simulink model "humanCarFollowerController_microscopic"  (R2016a)
settings: Solver=FixedStepAuto  StartTime=0.0  StopTime=inf  RelTol=1e-3
undefined symbols (not defined in the file or in its folder): Angular, Linear
libraries: robotlib x6
settings Model: Creator=ece446  LastModifiedBy=ece446
settings OptimizationCC: OptimizeModelRefInitCode=on  LifeSpan=Inf  MaxStackSize=64
settings HardwareCC: ProdBitPerInt=16  ProdBitPerPointer=16  ProdLargestAtomicFloat=None  ProdIntDivRoundTo=Undefined  ProdEndianess=Unspecified  ProdWordSize=16  ProdHWDeviceType=Generic->Unspecified (assume 32-bit Generic)  UseEmbeddedCoderFeatures=off
settings RTWCC: SystemTargetFile=ert.tlc  HardwareBoard=Robot Operating System (ROS)  TemplateMakefile=ert_default_tmf  GenerateReport=on  Toolchain=Catkin  IncludeHyperlinkInReport=on  LaunchReport=on  TargetLang=C++  GenerateTraceInfo=on  GenerateTraceReport=on  GenerateTraceReportSl=on  GenerateTraceReportSf=on  GenerateTraceReportEml=on
settings CodeAppCC: ForceParamTrailComments=on  IgnoreCustomStorageClasses=off  OperatorAnnotations=on  SimulinkDataObjDesc=on  SFDataObjDesc=on  MATLABFcnDesc=on  InsertBlockDesc=on  MATLABSourceComments=on
settings ERTTargetCC: SupportNonInlinedSFcns=on

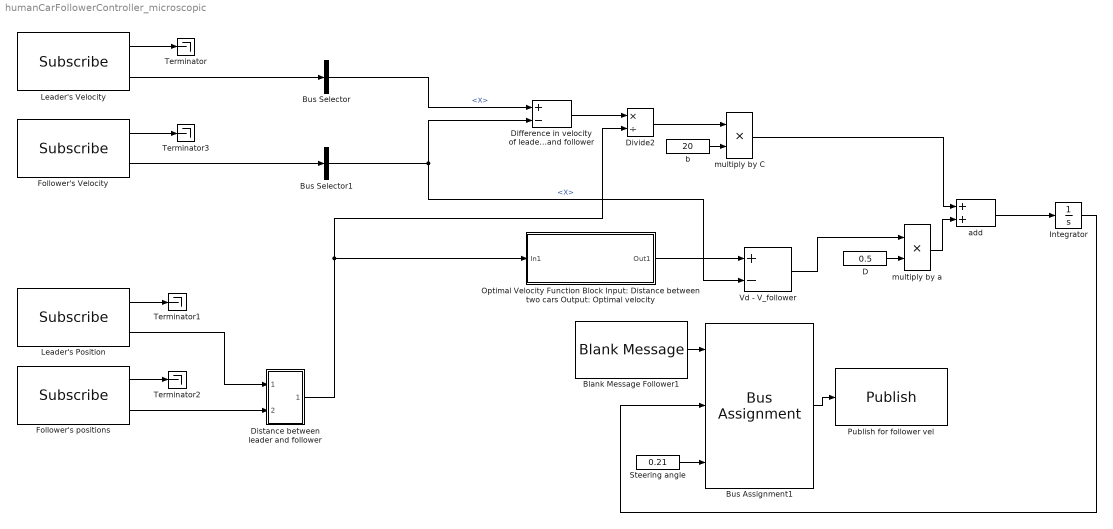
== system humanCarFollowerController_microscopic ==
  Blank Message Follower1 : robotlib/Blank Message  SourceLibraryInfo=This block requires Robotics System Toolbox  messageType=geometry_msgs/Twist  SampleTime=inf
  Bus Assignment1 : BusAssignment  AssignedSignals=Linear.X,Angular.Z
  Bus Selector : BusSelector  OutputSignals=Linear.X
  Bus Selector1 : BusSelector  OutputSignals=Linear.X
  D : Constant  Value=0.5
  "Difference in velocity of leader and follower " : Sum  Inputs=+-
  Distance between leader and follower : Subsystem
  Divide2 : Product  Inputs=*/
  Follower's Velocity : robotlib/Subscribe  SourceLibraryInfo=This block requires Robotics System Toolbox  topicSource=Specify your own  topic=/follower_sim/vel  messageType=geometry_msgs/Twist  sampleTime=-1  messageQueueLength=1
  Follower's positions : robotlib/Subscribe  SourceLibraryInfo=This block requires Robotics System Toolbox  topicSource=Select from ROS network  topic=/follower_sim/odom  messageType=nav_msgs/Odometry  sampleTime=-1  messageQueueLength=1
  Integrator : Integrator
  Leader's Position : robotlib/Subscribe  SourceLibraryInfo=This block requires Robotics System Toolbox  topicSource=Select from ROS network  topic=/azcar_sim/odom  messageType=nav_msgs/Odometry  sampleTime=-1  messageQueueLength=1
  Leader's Velocity : robotlib/Subscribe  SourceLibraryInfo=This block requires Robotics System Toolbox  topicSource=Select from ROS network  topic=/azcar_sim/vel  messageType=geometry_msgs/Twist  sampleTime=-1  messageQueueLength=1
  Optimal Velocity Function Block Input: Distance between two cars Output: Optimal velocity : Subsystem
  Publish for follower vel : robotlib/Publish  SourceLibraryInfo=This block requires Robotics System Toolbox  topicSource=Select from ROS network  topic=/follower_sim/cmd_vel  messageType=geometry_msgs/Twist  messageQueueLength=1
  Steering angle : Constant  Value=0.21
  Terminator{,1..3} (4 alike) : Terminator
  Vd - V_follower : Sum  Inputs=+-
  add : Sum
  b : Constant  Value=20
  "multiply by C " : Product
  multiply by a : Product
  wires:
  Blank Message Follower1/1 -> Bus Assignment1/1
  Bus Assignment1/1 -> Publish for follower vel/1
  Steering angle/1 -> Bus Assignment1/3
  Leader's Position/1 -> Terminator1/1
  Follower's positions/1 -> Terminator2/1
  Leader's Position/2 -> Distance between leader and follower/1(In1)
  Follower's positions/2 -> Distance between leader and follower/2(In2)
  Distance between leader and follower/1(Out1) -> Divide2/2, Optimal Velocity Function Block Input: Distance between two cars Output: Optimal velocity/1(In1)
  Leader's Velocity/2 -> Bus Selector/1
  Leader's Velocity/1 -> Terminator/1
  Bus Selector/1 -> "Difference in velocity of leader and follower "/1  "<X>"
  Follower's Velocity/2 -> Bus Selector1/1
  Follower's Velocity/1 -> Terminator3/1
  Bus Selector1/1 -> "Difference in velocity of leader and follower "/2, Vd - V_follower/2  "<X>"
  "Difference in velocity of leader and follower "/1 -> Divide2/1
  Divide2/1 -> "multiply by C "/1
  b/1 -> "multiply by C "/2
  Optimal Velocity Function Block Input: Distance between two cars Output: Optimal velocity/1(Out1) -> Vd - V_follower/1
  D/1 -> multiply by a/2
  Vd - V_follower/1 -> multiply by a/1
  "multiply by C "/1 -> add/1
  multiply by a/1 -> add/2
  add/1 -> Integrator/1
  Integrator/1 -> Bus Assignment1/2

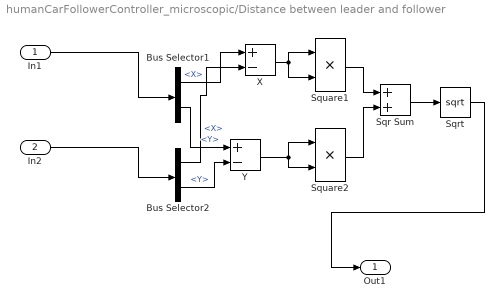
== system humanCarFollowerController_microscopic/Distance between leader and follower ==
  In1 : Inport
  In2 : Inport  Port=2
  Bus Selector1 : BusSelector  OutputSignals=Pose.Pose.Position.X,Pose.Pose.Position.Y
  Bus Selector2 : BusSelector  OutputSignals=Pose.Pose.Position.X,Pose.Pose.Position.Y
  Sqr Sum : Sum
  Sqrt : Sqrt  SaturateOnIntegerOverflow=on
  Square1 : Product
  Square2 : Product
  X : Sum  Inputs=+-
  Y : Sum  Inputs=+-
  Out1 : Outport
  wires:
  Bus Selector1/1 -> X/1  "<X>"
  Bus Selector2/2 -> Y/2  "<Y>"
  Square2/1 -> Sqr Sum/2
  Sqr Sum/1 -> Sqrt/1
  Square1/1 -> Sqr Sum/1
  Bus Selector1/2 -> Y/1  "<Y>"
  In1/1 -> Bus Selector1/1
  Bus Selector2/1 -> X/2  "<X>"
  Y/1 -> Square2/2, Square2/1
  X/1 -> Square1/2, Square1/1
  Sqrt/1 -> Out1/1
  In2/1 -> Bus Selector2/1

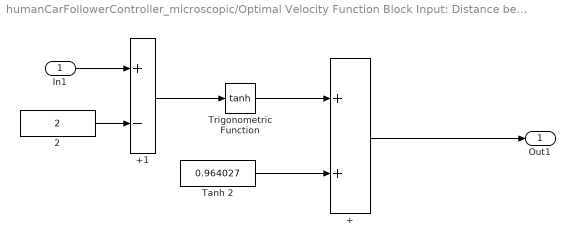
== system humanCarFollowerController_microscopic/Optimal Velocity Function Block Input: Distance between two cars Output: Optimal velocity ==
  In1 : Inport
  + : Sum
  +1 : Sum  Inputs=+-
  2 : Constant  Value=2
  Tanh 2 : Constant  Value=0.964027
  Trigonometric Function : Trigonometry  Operator=tanh
  Out1 : Outport
  wires:
  In1/1 -> +1/1
  2/1 -> +1/2
  +1/1 -> Trigonometric Function/1
  Trigonometric Function/1 -> +/1
  Tanh 2/1 -> +/2
  +/1 -> Out1/1
